simulink model "Model"  (R2016b)
settings: Solver=FixedStepAuto  StartTime=0.0  StopTime=t  FixedStep=Ts  RelTol=1e-3
model workspace (MAT data in the model file):
  index = Simulink.Signal
  index.DataType = 'double'
  index.Dimensions = 1
  index.DimensionsMode = 'Fixed'
  index.Complexity = 'real'
  index.SampleTime = -1
  index.SamplingMode = 'auto'
  index.InitialValue = '1'
values from neighbouring files (symbols this model uses):
  dx = 2.86    [Parameters.m]
  dy = 32.5    [Parameters.m]
  dyaw = 0.22285    [Parameters.m]
  F1 = fillin(time_base,time_F,F1temp)    [ExtractTopics.m]    (also in Verification.m = F1(105:end-100); dataTurn.mat = [-0.940797610436 -0.940797610436 -0.940797610436 -0.94079761; forces.mat = [-0.940797610436 -0.940797610436 -0.940797610436 -0.94079761)
  F2 = fillin(time_base,time_F,F2temp)    [ExtractTopics.m]    (also in Verification.m = F2(105:end-100); dataTurn.mat = [12.110592938 12.110592938 12.110592938 12.110592938 12.1105; forces.mat = [12.110592938 12.110592938 12.110592938 12.110592938 12.1105)
  Iz = 1.10675    [Parameters.m]
  l1 = 0.05    [Parameters.m]
  l2 = 0.05    [Parameters.m]
  m = 13    [Parameters.m]
  Ts = 0.05    [Parameters.m]    (also in Verification.m = t /samples)
  yaw_init = pi    (= 3.14159265359)    [Verification.m]
libraries: simulink x2
settings Model: Creator=USUARIO  LastModifiedBy=USUARIO
settings DataIOCC: Refine=100

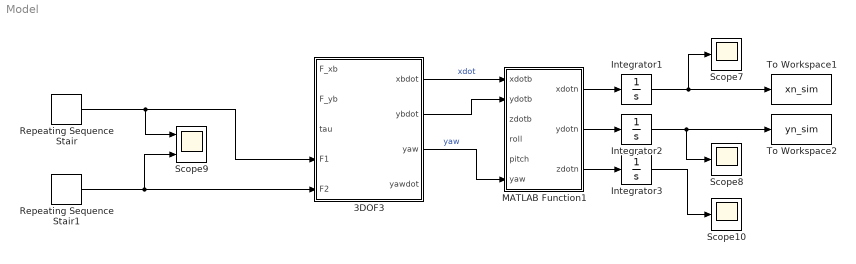
== system Model ==
  3DOF3 : Subsystem
  Integrator1 : Integrator
  Integrator2 : Integrator
  Integrator3 : Integrator
  MATLAB Function1 : MATLAB Function  TreatAsAtomicUnit=on
  Repeating Sequence Stair : simulink/Sources/Repeating Sequence Stair  OutValues=F1(115:203)  tsamp=Ts  OutMin=[]  OutMax=[]  OutDataTypeStr=double  OutputDataTypeScalingMode=double  OutDataType=fixdt(0,8)  ConRadixGroup=Best Precision: Vector-wise  OutScaling=2^-12
  Repeating Sequence Stair1 : simulink/Sources/Repeating Sequence Stair  OutValues=F2(115:203)  tsamp=Ts  OutMin=[]  OutMax=[]  OutDataTypeStr=double  OutputDataTypeScalingMode=double  OutDataType=fixdt(0,8)  ConRadixGroup=Best Precision: Vector-wise  OutScaling=2^-12
  Scope10 : Scope
  Scope7 : Scope
  Scope8 : Scope
  Scope9 : Scope  NumInputPorts=2
  To Workspace1 : ToWorkspace  VariableName=xn_sim  SaveFormat=Timeseries  SampleTime=-1
  To Workspace2 : ToWorkspace  VariableName=yn_sim  SaveFormat=Timeseries  SampleTime=-1
  wires:
  3DOF3/1(xbdot) -> MATLAB Function1/1(xdotb)  "xdot"
  3DOF3/2(ybdot) -> MATLAB Function1/2(ydotb)
  3DOF3/3(yaw) -> MATLAB Function1/6(yaw)  "yaw"
  Integrator1/1 -> To Workspace1/1, Scope7/1
  Integrator2/1 -> To Workspace2/1, Scope8/1
  MATLAB Function1/3(zdotn) -> Integrator3/1
  MATLAB Function1/1(xdotn) -> Integrator1/1
  MATLAB Function1/2(ydotn) -> Integrator2/1
  Integrator3/1 -> Scope10/1
  Repeating Sequence Stair1/1 -> Scope9/2, 3DOF3/5(F2)
  Repeating Sequence Stair/1 -> 3DOF3/4(F1), Scope9/1

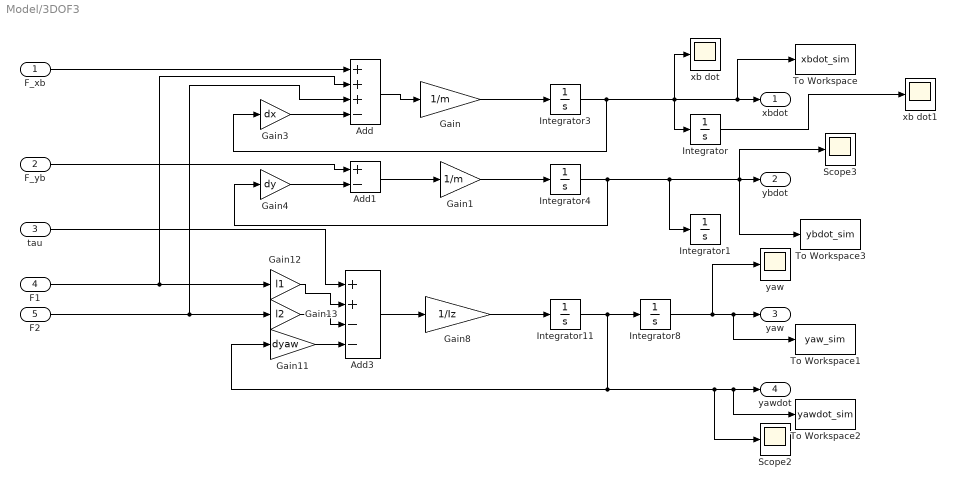
== system Model/3DOF3 ==
  F_xb : Inport
  F_yb : Inport  Port=2
  tau : Inport  Port=3
  F1 : Inport  Port=4
  F2 : Inport  Port=5
  Add : Sum  Inputs=+++-
  Add1 : Sum  Inputs=+-
  Add3 : Sum  Inputs=++--
  Gain : Gain  Gain=1/m
  Gain1 : Gain  Gain=1/m
  Gain11 : Gain  Gain=dyaw
  Gain12 : Gain  Gain=l1
  Gain13 : Gain  Gain=l2
  Gain3 : Gain  Gain=dx
  Gain4 : Gain  Gain=dy
  Gain8 : Gain  Gain=1/Iz
  Integrator{,1,3..4,11} (5 alike) : Integrator
  Integrator8 : Integrator  InitialCondition=yaw_init
  Scope2 : Scope
  Scope3 : Scope
  To Workspace : ToWorkspace  VariableName=xbdot_sim  SaveFormat=Timeseries  SampleTime=Ts
  To Workspace1 : ToWorkspace  VariableName=yaw_sim  SaveFormat=Timeseries  SampleTime=Ts
  To Workspace2 : ToWorkspace  VariableName=yawdot_sim  SaveFormat=Timeseries  SampleTime=Ts
  To Workspace3 : ToWorkspace  VariableName=ybdot_sim  SaveFormat=Timeseries  SampleTime=Ts
  xb dot : Scope
  xb dot1 : Scope
  "yaw " : Scope
  xbdot : Outport
  ybdot : Outport  Port=2
  yaw : Outport  Port=3
  yawdot : Outport  Port=4
  wires:
  tau/1 -> Add3/1
  F_xb/1 -> Add/1
  F_yb/1 -> Add1/1
  Add1/1 -> Gain1/1
  F2/1 -> Gain13/1, Add/3
  F1/1 -> Gain12/1, Add/2
  Integrator8/1 -> yaw/1, To Workspace1/1, "yaw "/1
  Integrator4/1 -> Scope3/1, ybdot/1, To Workspace3/1, Integrator1/1, Gain4/1
  Integrator3/1 -> Gain3/1, xbdot/1, To Workspace/1, Integrator/1, xb dot/1
  Gain13/1 -> Add3/3
  Gain11/1 -> Add3/4
  Add3/1 -> Gain8/1
  Gain12/1 -> Add3/2
  Gain/1 -> Integrator3/1
  Add/1 -> Gain/1
  Gain3/1 -> Add/4
  Gain1/1 -> Integrator4/1
  Gain4/1 -> Add1/2
  Gain8/1 -> Integrator11/1
  Integrator11/1 -> Integrator8/1, Gain11/1, To Workspace2/1, yawdot/1, Scope2/1
  Integrator/1 -> xb dot1/1

== matlab function Model/MATLAB Function1 ==
  data: xdotb input; xdotn output; ydotb input; zdotb input; roll input; pitch input; yaw input; ydotn output; zdotn output
function [xdotn,ydotn,zdotn] = fcn(xdotb,ydotb,zdotb,roll,pitch,yaw)
R=[cos(pitch)*cos(yaw) sin(roll)*sin(pitch)*cos(yaw)-cos(roll)*sin(yaw) ...
                          cos(roll)*sin(pitch)*cos(yaw)+sin(roll)*sin(yaw);
   cos(pitch)*sin(yaw) sin(roll)*sin(pitch)*sin(yaw)+cos(roll)*cos(yaw) ...
                          cos(roll)*sin(pitch)*sin(yaw)-sin(roll)*cos(yaw);
   -sin(pitch) sin(roll)*cos(pitch) cos(roll)*cos(pitch)];

n=R*[xdotb;ydotb;zdotb];

xdotn=n(1);
ydotn=n(2);
zdotn=n(3);
end
